simulink model "CAD_exp2_10"  (R2019a)
settings: Solver=VariableStepAuto  StartTime=0.0  StopTime=60  RelTol=1e-3
settings Model: Creator=83621  LastModifiedBy=83621

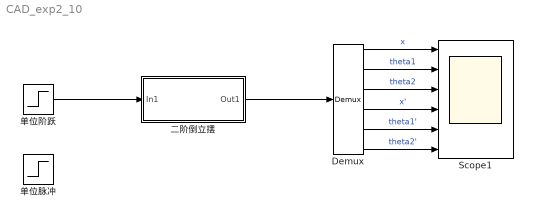
== system CAD_exp2_10 ==
  Demux : Demux  Outputs=6
  Scope1 : Scope  NumInputPorts=6
  二阶倒立摆 : Subsystem  mask{m0=1.32, m1=0.132, m2=0.04, j1=0.0036, j2=0.004, l1=0.27, l2=0.09, l=0.18, f0=6.7697, f1=0.0007056, f2=0.0007056, g0=1, g=9.8}
      mask DialogControl name1 Prompt: name1
  单位脉冲 : Step  Time=0.01  Before=100  After=0  SampleTime=0
  单位阶跃 : Step  SampleTime=0
  wires:
  二阶倒立摆/1(Out1) -> Demux/1
  Demux/4 -> Scope1/4  "x'"
  Demux/3 -> Scope1/3  "theta2"
  Demux/2 -> Scope1/2  "theta1"
  Demux/1 -> Scope1/1  "x"
  Demux/5 -> Scope1/5  "theta1'"
  Demux/6 -> Scope1/6  "theta2'"
  单位阶跃/1 -> 二阶倒立摆/1(In1)

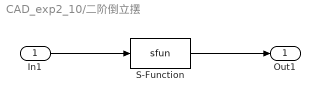
== system CAD_exp2_10/二阶倒立摆 ==
  In1 : Inport
  S-Function : S-Function  FunctionName=sfun  Parameters=m0,m1,m2,j1,j2,l1,l2,l,f0,f1,f2,g0,g  SFunctionDeploymentMode=off  EnableBusSupport=off
  Out1 : Outport
  wires:
  In1/1 -> S-Function/1
  S-Function/1 -> Out1/1
